simulink model "stepperXploer"  (R2025b)
settings: Solver=FixedStepAuto  StartTime=0.0  StopTime=inf  FixedStep=0.001  RelTol=1e-3
values from neighbouring files (symbols this model uses):
  frequency = frequency(1:min_len)    [openSplitAndEachPlot_Freq.m]    (also in untitled3.m; untitled9.m)
  n = DS.numElements    [spiltefile.m]
undefined symbols (not defined in the file or in its folder): Blocking, LF, Non
libraries: amg_usbconverter_n_connect_lib x3, dspfdesign x2, dspstat3 x1, waijung_addon_module x1
settings Model: Creator=beamk  LastModifiedBy=Asus

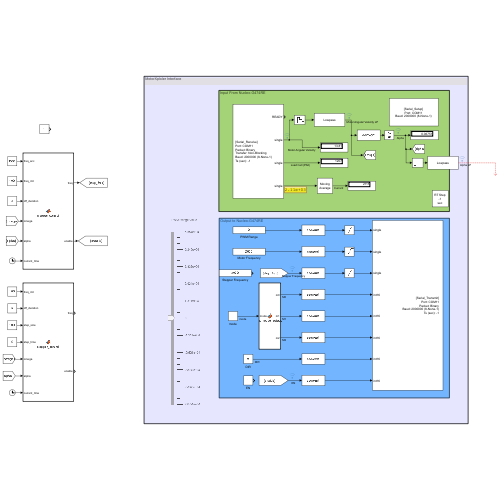
[thumbnail: Simulink's stored preview of the top-level diagram]
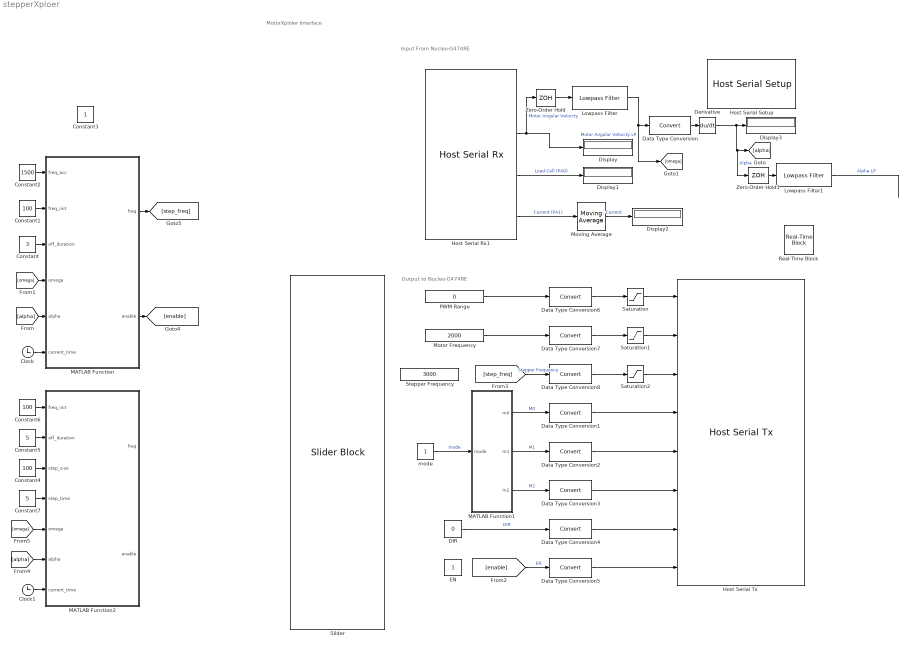
== system stepperXploer ==
  note: Output to Nucleo-G474RE
  note: Input From Nucleo-G474RE
  note: MotorXploler Interface
  Clock : Clock
  Clock1 : Clock
  Constant : Constant  Value=3
  Constant1 : Constant  Value=100
  Constant2 : Constant  Value=1500
  Constant3 : Constant
  Constant4 : Constant  Value=100
  Constant5 : Constant  Value=5
  Constant6 : Constant  Value=100
  Constant7 : Constant  Value=5
  DIR : Constant  Value=0
  Data Type Conversion{,1..8} (9 alike) : DataTypeConversion  SaturateOnIntegerOverflow=off  RndMeth=Floor
  Derivative : Derivative
  Display{,1..3} (4 alike) : Display
  EN : Constant
  Host Serial Rx1 : amg_usbconverter_n_connect_lib/Host Serial Rx  conf=rx  port=<auto>  baudrate=2000000  databits=8  parity=None  stopbit=1  flowcontrol=None  transfer=Non-Blocking  timeout=5  packetmode=Binary  enableinitialvalues=off  initialvalues=[]  binheader='25'  binterminator='4E'  porttype_double=0  porttype_single=3  porttype_int8=0  porttype_uint8=0  porttype_int16=0  porttype_uint16=0  porttype_int32=0  porttype_uint32=0  asciiformat='%f,%f,%d,%d'  rx_asciiterminator="LF (0x0A - \"\\n\")"  tx_asciiterminator="CRLF (0x0D 0x0A - \"\\r\\n\")"  sampletime=-1  enablecustomportlabel=off  cinputportlabel=0  coutputportlabel=A  portpinstr=0  blockid=HostSerialRx1  inputporttype=[]  inputportwidth=[]  inputportlabel={}  outputporttype=[3 1 1 1]  outputportwidth=[1 1 1 1]  outputportlabel={'READY','single','single','single'}  compat=0  optionstring=[]  autoport='COM11'
  Host Serial Setup : amg_usbconverter_n_connect_lib/Host Serial Setup  conf=setup  port=<auto>  baudrate=2000000  databits=8  parity=None  stopbit=1  flowcontrol=None  transfer=Blocking  timeout=2  packetmode=Binary  initialvalues=[]  binheader='7E 7E'  binterminator='03 03'  porttype_double=0  porttype_single=1  porttype_int8=0  porttype_uint8=0  porttype_int16=0  porttype_uint16=0  porttype_int32=0  porttype_uint32=2  asciiformat='%d %u %x'  rx_asciiterminator="CRLF (0x0D 0x0A - \"\\r\\n\")"  tx_asciiterminator="CRLF (0x0D 0x0A - \"\\r\\n\")"  sampletime=-1  enablecustomportlabel=off  cinputportlabel=0  coutputportlabel=A  portpinstr=0  blockid=HostSerialSetup  inputporttype=[]  inputportwidth=[]  inputportlabel={}  outputporttype=[]  outputportwidth=[]  outputportlabel={}  compat=0  optionstring=[]  autoport='COM11'
  Host Serial Tx : amg_usbconverter_n_connect_lib/Host Serial Tx  conf=tx  port=<auto>  baudrate=2000000  databits=8  parity=None  stopbit=1  flowcontrol=None  transfer=Blocking  timeout=2  packetmode=Binary  initialvalues=[]  binheader='25'  binterminator='4E'  porttype_double=0  porttype_single=3  porttype_int8=0  porttype_uint8=0  porttype_int16=5  porttype_uint16=0  porttype_int32=0  porttype_uint32=0  asciiformat='%d,%f'  rx_asciiterminator="CRLF (0x0D 0x0A - \"\\r\\n\")"  tx_asciiterminator="CRLF (0x0D 0x0A - \"\\r\\n\")"  sampletime=-1  enablecustomportlabel=off  cinputportlabel=0  coutputportlabel=A  portpinstr=0  blockid=HostSerialTx  inputporttype=[1 1 1 4 4 4 4 4]  inputportwidth=[1 1 1 1 1 1 1 1]  inputportlabel={'single','single','single','int16','int16','int16','int16','int16'}  outputporttype=[]  outputportwidth=[]  outputportlabel={}  compat=0  optionstring=[]  autoport='COM11'
      settings: SourceProductName=aMG USB Converter N
  Lowpass Filter : dspfdesign/Lowpass Filter  FilterType=FIR  DesignForMinimumOrder=on  FilterOrder=50  PassbandFrequency=0.02  StopbandFrequency=0.04  PassbandRipple=0.1  StopbandAttenuation=80  SampleRateMode=Use normalized frequency (0 to 1)  SampleRate=44100  SimulateUsing=Interpreted execution  roundingMode=Floor  coeffsDataTypeStr=fixdt(1,16)
  Lowpass Filter1 : dspfdesign/Lowpass Filter  FilterType=FIR  DesignForMinimumOrder=on  FilterOrder=50  PassbandFrequency=0.01  StopbandFrequency=0.02  PassbandRipple=0.1  StopbandAttenuation=80  SampleRateMode=Use normalized frequency (0 to 1)  SampleRate=44100  SimulateUsing=Interpreted execution  roundingMode=Floor  coeffsDataTypeStr=fixdt(1,16)
  MATLAB Function : MATLAB Function  TreatAsAtomicUnit=on
  MATLAB Function1 : MATLAB Function  TreatAsAtomicUnit=on
  MATLAB Function2 : MATLAB Function  TreatAsAtomicUnit=on
  Motor Frequency : Constant  Value=2000  OutDataTypeStr=single
  Moving Average : dspstat3/Moving Average  Method=Sliding window  ForgettingFactorPort=off  SpecifyWindowLength=on  WindowLength=11  OverlapLength=10  AllowArbitraryInputLength=off  ForgettingFactor=0.9  SimulateUsing=Interpreted execution
  PWM Range : Constant  Value=0  OutDataTypeStr=single
  Real-Time Block : waijung_addon_module/Real-Time Block  Priority=0  setting=Default  sampletime=-1
      settings: SourceProductName=Misc
  Saturation : Saturate  UpperLimit=65535  LowerLimit=-65535
  Saturation1 : Saturate  UpperLimit=20000  LowerLimit=0
  Saturation2 : Saturate  UpperLimit=inf  LowerLimit=0
  Slider : SliderBlock  ScaleMin=-65535  ScaleMax=65535
  Stepper Frequency : Constant  Value=3000  OutDataTypeStr=single
  Zero-Order Hold : ZeroOrderHold  SampleTime=-1
  Zero-Order Hold1 : ZeroOrderHold  SampleTime=-1
  mode : Constant
  wires:
  Host Serial Rx1/2 -> Display/1, Zero-Order Hold/1  "Motor Angular Velocity"
  Host Serial Rx1/3 -> Display1/1  "Load Cell (PA0)"
  MATLAB Function1/1(m0) -> Data Type Conversion1/1  "M0"
  DIR/1 -> Data Type Conversion4/1  "DIR"
  MATLAB Function1/2(m1) -> Data Type Conversion2/1  "M1"
  MATLAB Function1/3(m2) -> Data Type Conversion3/1  "M2"
  Motor Frequency/1 -> Data Type Conversion7/1
  Data Type Conversion1/1 -> Host Serial Tx/4
  Data Type Conversion2/1 -> Host Serial Tx/5
  Data Type Conversion3/1 -> Host Serial Tx/6
  Data Type Conversion4/1 -> Host Serial Tx/7
  Data Type Conversion5/1 -> Host Serial Tx/8
  Data Type Conversion6/1 -> Saturation/1
  Saturation/1 -> Host Serial Tx/1
  Data Type Conversion7/1 -> Saturation1/1
  Data Type Conversion8/1 -> Saturation2/1
  PWM Range/1 -> Data Type Conversion6/1
  Saturation1/1 -> Host Serial Tx/2
  Saturation2/1 -> Host Serial Tx/3
  Host Serial Rx1/4 -> Moving Average/1  "Current (PA1)"
  Derivative/1 -> Zero-Order Hold1/1, [alpha], Display3/1  "Alpha"
  Lowpass Filter/1 -> [omega], Data Type Conversion/1  "Motor Angular Velocity LP"
  Data Type Conversion/1 -> Derivative/1
  Zero-Order Hold/1 -> Lowpass Filter/1
  [alpha] -> MATLAB Function/5(alpha)
  [omega] -> MATLAB Function/4(omega)
  Constant/1 -> MATLAB Function/3(off_duration)
  Constant1/1 -> MATLAB Function/2(freq_init)
  Constant2/1 -> MATLAB Function/1(freq_acc)
  Clock/1 -> MATLAB Function/6(current_time)
  [enable] -> Data Type Conversion5/1  "EN"
  [step_freq] -> Data Type Conversion8/1  "Stepper Frequency"
  mode/1 -> MATLAB Function1/1(mode)  "mode"
  Zero-Order Hold1/1 -> Lowpass Filter1/1
  Lowpass Filter1/1 -> ?  "Alpha LP"
  Clock1/1 -> MATLAB Function2/7(current_time)
  [alpha] -> MATLAB Function2/6(alpha)
  [omega] -> MATLAB Function2/5(omega)
  Constant6/1 -> MATLAB Function2/1(freq_init)
  Constant5/1 -> MATLAB Function2/2(off_duration)
  Constant4/1 -> MATLAB Function2/3(step_size)
  Constant7/1 -> MATLAB Function2/4(step_time)
  MATLAB Function/1(freq) -> [step_freq]
  Moving Average/1 -> Display2/1  "Current"
  MATLAB Function/2(enable) -> [enable]

== matlab function stepperXploer/MATLAB Function1 ==
  data: mode input; m0 output; m1 output; m2 output
function [m0, m1, m2] = step_mode_selector(mode)
% mode = 1,2,4,8,16,32

m0 = 0;
m1 = 0;
m2 = 0;

switch mode
    case 1      % Full step
        m2 = 0; m1 = 0; m0 = 0;

    case 2      % Half step
        m2 = 0; m1 = 0; m0 = 1;

    case 4      % 1/4 step
        m2 = 0; m1 = 1; m0 = 0;

    case 8      % 1/8 step
        m2 = 0; m1 = 1; m0 = 1;

    case 16     % 1/16 step
        m2 = 1; m1 = 0; m0 = 0;

    case 32     % 1/32 step
        m2 = 1; m1 = 0; m0 = 1;

    otherwise   % ค่าไม่ถูกต้องให้ full step
        m2 = 0; m1 = 0; m0 = 0;
end

== matlab function stepperXploer/MATLAB Function ==
  data: freq_acc input; freq output; freq_init input; off_duration input; omega input; alpha input; current_time input; enable output
function [freq, enable] = stepper_control(freq_acc, freq_init, off_duration, omega, alpha, current_time)
%#codegen

% Persistent states
persistent state start_time current_freq
if isempty(state)
    state = 0;             % 0 = off phase, 1 = accel phase
    start_time = 0;
    current_freq = 100;
end

freq = 0;
enable = 1;
dt = current_time - start_time;
current_freq = freq_init + freq_acc * dt;
switch state
    case 0
        % Off phase
        enable = 1;
        freq = 0;

        if current_time - start_time >= off_duration
            % Switch to accel mode
            state = 1;
            current_freq = freq_init;
            start_time = current_time;
        end

    case 1
        % Acceleration phase
        enable = 0;

        % Linear or custom acceleration
        dt = current_time - start_time;
        current_freq = freq_init + freq_acc * dt;

        freq = current_freq;

        % Motor stop condition
        if alpha <= -1500 && omega <= abs(5) || (current_freq > 1000 && omega < abs(0.2))
            % Reset cycle
            state = 0;
            start_time = current_time;
            freq = 0;
            enable = 1;
        end
end

== matlab function stepperXploer/MATLAB Function2 ==
  data: freq output; freq_init input; off_duration input; enable output; step_size input; step_time input; omega input; alpha input; current_time input
function [freq, enable] = stepper_control(freq_init, off_duration, step_size, step_time, omega, alpha, current_time)
%#codegen

persistent state start_time current_freq last_step_time
if isempty(state)
    state = 0;                % 0 = off, 1 = stepping
    start_time = 0;
    current_freq = 0;
    last_step_time = 0;
end

freq = 0;
enable = 1;

switch state
    case 0
        % Off phase
        enable = 1;
        freq = 0;

        if current_time - start_time >= off_duration
            state = 1;
            current_freq = freq_init;
            last_step_time = current_time;
            start_time = current_time;
        end

    case 1
        % Step-based frequency ramp
        enable = 0;

        % ทำ step เมื่อถึงเวลา
        if (current_time - last_step_time) >= step_time
            current_freq = current_freq + step_size;
            last_step_time = current_time;
        end

        freq = current_freq;

        % Stop condition (ตามที่คุณใช้เดิม)
        if (alpha <= -1500 && omega <= abs(5)) || ...
           (current_freq > 1000 && omega < abs(0.2))

            state = 0;
            start_time = current_time;
            enable = 1;
            freq = 0;
        end
end
